simulink model "P5_Ex19"  (R2018a)
settings: Solver=VariableStepAuto  StartTime=0.0  StopTime=Total_time  RelTol=1e-3
PreLoadFcn:
  |     K0=0.82/0.017;
  |     tau0=0.26;
  |     % modelització del sistema a partir de les seves característiques
  |     N=9;
  |     Kpot=1.62;
  |     planta=tf([K0],[tau0 1]);
  |     conversor=tf([1],[N 0]);
  |     potenciometre=tf([Kpot],[1]);
  | 
  |     % modelització en temps continu
  |     sistema_continu=planta*conversor*potenciometre;
  |     Ts=0.005;
  |     zc=1;
  |     zp=1;
  |     k=1;
  |     Total_time=20;
  |     % repeticions
  |     N=2.5;
  |     T_ona=Total_time/N;
  |     Ts_dif=1.0000e-003;
  |     Ts=0.01;
  |     i=1;
  |     Vmax=3;
  |     Vmin=-3;
  |     input_vector=[Vmax Vmin];
  |     while (i<=N)
  |         input_vector=[input_vector [Vmax Vmin]];
  |         i=i+1;
  |     end
libraries: simulink x2
settings Model: Creator=Eneko Lerma  LastModifiedBy=Eneko Lerma

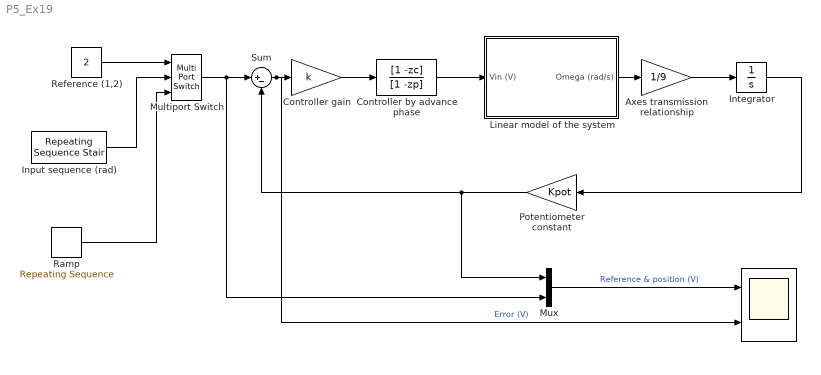
== system P5_Ex19 ==
  "  " : Scope  NumInputPorts=2
  "Axes transmission relationship " : Gain  Gain=1/9
  Controller by advance phase : DiscreteTransferFcn  Numerator=[1 -zc]  Denominator=[1 -zp]  SampleTime=Ts
  Controller gain : Gain  Gain=k
  Input sequence (rad) : simulink/Sources/Repeating Sequence Stair  OutValues=input_vector  tsamp=T_ona/2  OutMin=[]  OutMax=[]  OutDataTypeStr=float('double')  OutputDataTypeScalingMode=Specify via dialog  OutDataType=float('double')  ConRadixGroup=Best Precision: Vector-wise  OutScaling=2^-12
  Integrator : Integrator
  Linear model of the system : Subsystem
  Multiport Switch : MultiPortSwitch  Inputs=2
  Mux : Mux  Inputs=2
  Potentiometer constant : Gain  Gain=Kpot
  Ramp : simulink/Sources/Repeating Sequence  rep_seq_t="[0    0.1000    0.2000    0.3000    0.4000    0.5000    0.6000    0.7000    0.8000 0.9000    1.0000    1.1000    1.2000    1.3000    1.4000    1.5000    1.6000    1.7000 1.8000    1.9000    2.0000    2.1000    2.2000    2.3000    2.4000    2.5000    2.6000 2.7000    2.8000    2.9000    3.0000    3.1000    3.2000    3.3000    3.4000    3.5000\t3.6000    3.7000    3.8000    3.9000    4.0000    4.1000    4.2000    4.3000    4.4000    4.5000    4.6000    4.7000    4.8000    4.9000    5.0000]"  rep_seq_y=[-2.0000,-1.9200,-1.8400,-1.7600,-1.6800,-1.6000,-1.5200,-1.4400,-1.3600,-1.2800,-1.2000,-1.1200,-1.0400,-0.9600,-0.8800,-0.8000,-0.7200,-0.6400,-0.5600,-0.4800,-0.4000,-0.3200,-0.2400,-0.1600,-0.0800,0,0.0800,0.1600,0.2400,0.3200,0.4000,0.4800,0.5600,0.6400,0.7200,0.8000,0.8800,0.9600,1.0400,1.1200,1.2000,1.2800,1.3600,1.4400,1.5200,1.6000,1.6800,1.7600,1.8400,1.9200,2.0000]
  Reference (1,2) : Constant  Value=2
  Sum : Sum  Inputs=|+-
  wires:
  Integrator/1 -> Potentiometer constant/1
  Reference (1,2)/1 -> Multiport Switch/1
  Sum/1 -> "  "/2, Controller gain/1  "Error (V)"
  Ramp/1 -> Multiport Switch/3
  Mux/1 -> "  "/1  "Reference & position (V)"
  Input sequence (rad)/1 -> Multiport Switch/2
  Controller by advance phase/1 -> Linear model of the system/1(Vin (V))
  Multiport Switch/1 -> Sum/1, Mux/2
  Potentiometer constant/1 -> Sum/2, Mux/1
  Linear model of the system/1(Omega (rad/s)) -> "Axes transmission relationship "/1
  Controller gain/1 -> Controller by advance phase/1
  "Axes transmission relationship "/1 -> Integrator/1

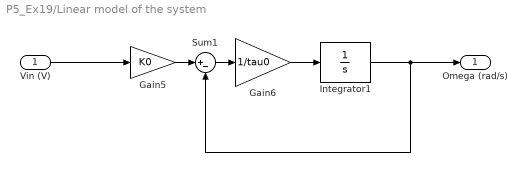
== system P5_Ex19/Linear model of the system ==
  Vin (V) : Inport
  Gain5 : Gain  Gain=K0
  Gain6 : Gain  Gain=1/tau0
  Integrator1 : Integrator
  Sum1 : Sum  Inputs=|+-
  Omega (rad/s) : Outport
  wires:
  Gain6/1 -> Integrator1/1
  Gain5/1 -> Sum1/1
  Sum1/1 -> Gain6/1
  Vin (V)/1 -> Gain5/1
  Integrator1/1 -> Omega (rad/s)/1, Sum1/2
